simulink model "signal_gain_control"  (R2022a)
settings: Solver=VariableStepAuto  StartTime=0.0  StopTime=10.0  RelTol=1e-3
settings Model: Creator=Laptop-Academy.com  LastModifiedBy=Laptop-Academy.com

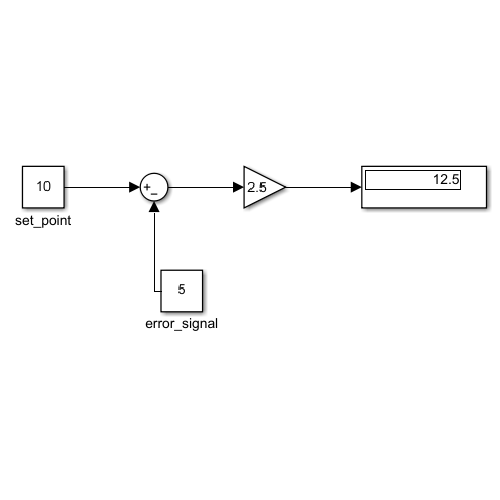
[thumbnail: Simulink's stored preview of the top-level diagram]
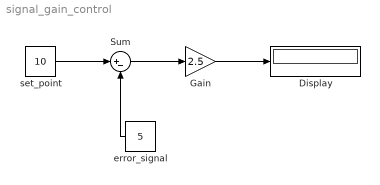
== system signal_gain_control ==
  Display : Display
  Gain : Gain  Gain=2.5
  Sum : Sum  Inputs=|+-
  error_signal : Constant  Value=5
  set_point : Constant  Value=10
  wires:
  set_point/1 -> Sum/1
  Sum/1 -> Gain/1
  error_signal/1 -> Sum/2
  Gain/1 -> Display/1
